simulink model "dynamic_simulation"  (R2020a)
settings: Solver=ode3  StartTime=0.0  StopTime=inf  FixedStep=0.01  RelTol=1e-3
undefined symbols (not defined in the file): name_max_length
libraries: robotlib x23, robotmaniplib x1
settings Model: Creator=ROS_PO  LastModifiedBy=paolo
settings OptimizationCC: EnhancedBackFolding=on  PassReuseOutputArgsAs=Individual arguments  ZeroExternalMemoryAtStartup=off  ZeroInternalMemoryAtStartup=off  MaxStackSize=64  OptimizeBlockOrder=speed  DifferentSizesBufferReuse=on  OptimizationCustomize=off  EfficientTunableParamExpr=on
settings DebuggingCC: ParameterTunabilityLossMsg=error
settings HardwareCC: ProdBitPerPointer=32  ProdBitPerSizeT=32  ProdBitPerPtrDiffT=32  ProdLargestAtomicFloat=None  ProdIntDivRoundTo=Undefined  ProdEndianess=Unspecified  ProdWordSize=32  ProdHWDeviceType=Generic->Unspecified (assume 32-bit Generic)
settings RTWCC: SystemTargetFile=ert.tlc  HardwareBoard=Robot Operating System (ROS)  TemplateMakefile=ert_default_tmf  GenerateReport=on  Toolchain=Catkin  IncludeHyperlinkInReport=on  LaunchReport=on  TargetLang=C++  GenerateTraceInfo=on  GenerateTraceReport=on  GenerateTraceReportSl=on  GenerateTraceReportSf=on  GenerateTraceReportEml=on
settings CodeAppCC: ForceParamTrailComments=on  IgnoreCustomStorageClasses=off  OperatorAnnotations=on  SimulinkDataObjDesc=on  SFDataObjDesc=on  InsertBlockDesc=on
settings ERTTargetCC: SupportContinuousTime=on  SupportVariableSizeSignals=on

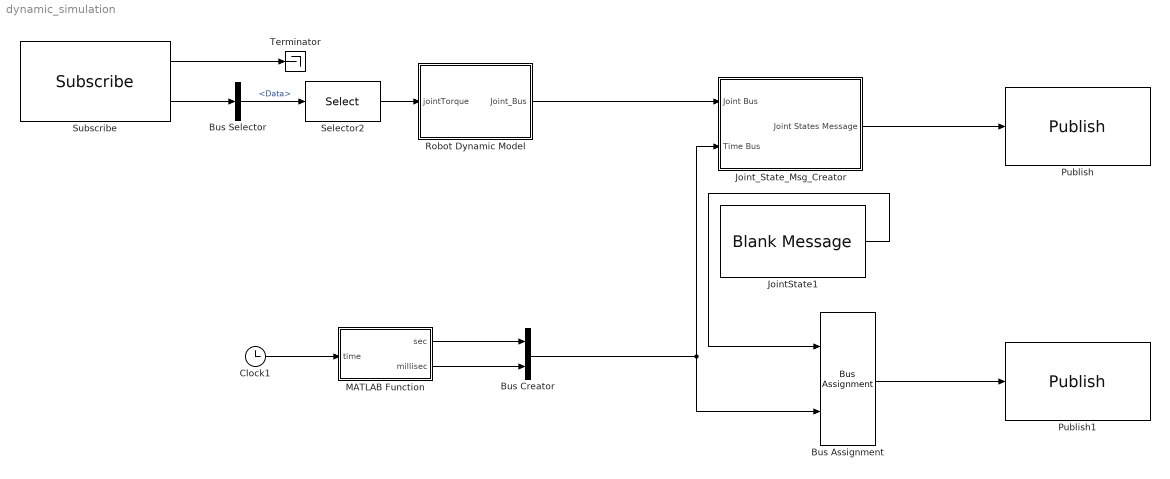
== system dynamic_simulation ==
  Bus Assignment : BusAssignment  AssignedSignals=Clock_
  Bus Creator : BusCreator  Inputs=2
  Bus Selector : BusSelector  OutputSignals=Data
  Clock1 : Clock
  JointState1 : robotlib/Blank Message  messageClass=Message  entityType=rosgraph_msgs/Clock  messageType=rosgraph_msgs/Clock  SampleTime=inf
  Joint_State_Msg_Creator : Subsystem
  MATLAB Function : MATLAB Function  TreatAsAtomicUnit=on
  Publish : robotlib/Publish  topicSource=Specify your own  topic=/joint_states  messageType=sensor_msgs/JointState  messageQueueLength=1
  Publish1 : robotlib/Publish  topicSource=Specify your own  topic=/clock  messageType=rosgraph_msgs/Clock  messageQueueLength=1
  Robot Dynamic Model : Subsystem
  Selector2 : Selector  IndexOptions=Starting index (dialog)  Indices=1  OutputSizes=6
  Subscribe : robotlib/Subscribe  topicSource=Specify your own  topic=/joint_torque  messageType=std_msgs/Float64MultiArray  sampleTime=-1  messageQueueLength=1
  Terminator : Terminator
  wires:
  Subscribe/1 -> Terminator/1
  Subscribe/2 -> Bus Selector/1
  Robot Dynamic Model/1(Joint_Bus) -> Joint_State_Msg_Creator/1(Joint Bus)
  Bus Selector/1 -> Selector2/1  "<Data>"
  MATLAB Function/1(sec) -> Bus Creator/1
  MATLAB Function/2(millisec) -> Bus Creator/2
  Clock1/1 -> MATLAB Function/1(time)
  Bus Creator/1 -> Bus Assignment/2, Joint_State_Msg_Creator/2(Time Bus)
  JointState1/1 -> Bus Assignment/1
  Bus Assignment/1 -> Publish1/1
  Joint_State_Msg_Creator/1(Joint States Message) -> Publish/1
  Selector2/1 -> Robot Dynamic Model/1(jointTorque)

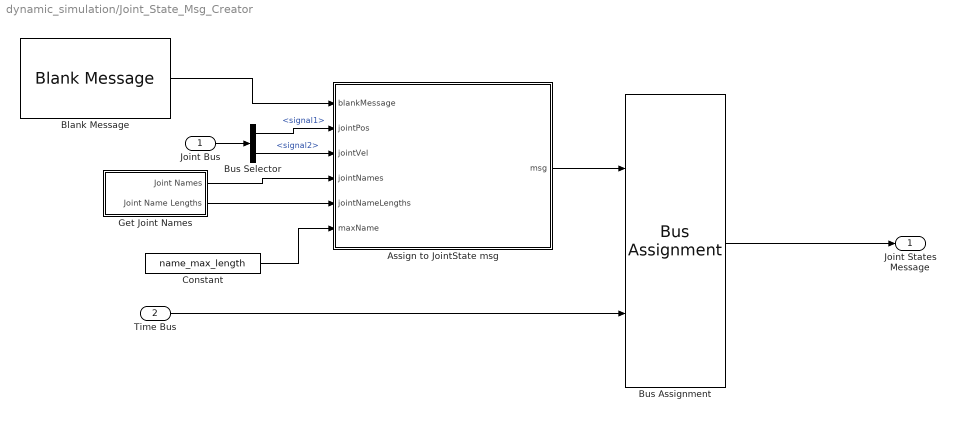
== system dynamic_simulation/Joint_State_Msg_Creator ==
  Joint Bus : Inport
  Time Bus : Inport  Port=2
  Assign to JointState msg : MATLAB Function  TreatAsAtomicUnit=on
  Blank Message : robotlib/Blank Message  messageClass=Message  entityType=sensor_msgs/JointState  messageType=sensor_msgs/JointState  SampleTime=inf
  Bus Assignment : BusAssignment  AssignedSignals=Header.Stamp
  Bus Selector : BusSelector  OutputSignals=signal1,signal2
  Constant : Constant  Value=name_max_length
  Get Joint Names : Subsystem
  Joint States Message : Outport
  wires:
  Joint Bus/1 -> Bus Selector/1
  Bus Selector/1 -> Assign to JointState msg/2(jointPos)  "<signal1>"
  Bus Selector/2 -> Assign to JointState msg/3(jointVel)  "<signal2>"
  Time Bus/1 -> Bus Assignment/2
  Bus Assignment/1 -> Joint States Message/1
  Blank Message/1 -> Assign to JointState msg/1(blankMessage)
  Assign to JointState msg/1(msg) -> Bus Assignment/1
  Get Joint Names/1(Joint Names) -> Assign to JointState msg/4(jointNames)
  Get Joint Names/2(Joint Name Lengths) -> Assign to JointState msg/5(jointNameLengths)
  Constant/1 -> Assign to JointState msg/6(maxName)

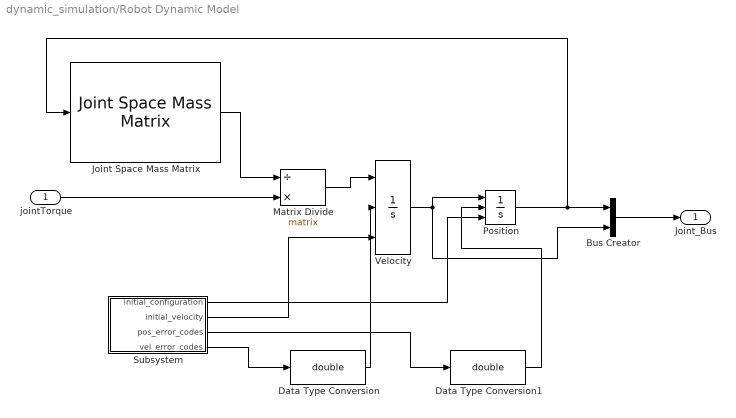
== system dynamic_simulation/Robot Dynamic Model ==
  jointTorque : Inport
  Bus Creator : BusCreator  Inputs=2
  Data Type Conversion : DataTypeConversion  OutDataTypeStr=double
  Data Type Conversion1 : DataTypeConversion  OutDataTypeStr=double
  Joint Space Mass Matrix : robotmaniplib/Joint Space Mass Matrix  RigidBodyTree=robot  SimulateUsing=Interpreted execution
  Matrix Divide : Product  Inputs=/*  Multiplication=Matrix(*)
  Position : Integrator  ExternalReset=falling  InitialConditionSource=external
  Subsystem : Subsystem
  Velocity : Integrator  ExternalReset=falling  InitialConditionSource=external
  Joint_Bus : Outport
  wires:
  Position/1 -> Joint Space Mass Matrix/1, Bus Creator/1
  Velocity/1 -> Position/1, Bus Creator/2
  Bus Creator/1 -> Joint_Bus/1
  Joint Space Mass Matrix/1 -> Matrix Divide/1
  jointTorque/1 -> Matrix Divide/2
  Matrix Divide/1 -> Velocity/1
  Subsystem/4(vel_error_codes) -> Data Type Conversion/1
  Subsystem/3(pos_error_codes) -> Data Type Conversion1/1
  Data Type Conversion/1 -> Velocity/2
  Subsystem/2(initial_velocity) -> Velocity/3
  Data Type Conversion1/1 -> Position/2
  Subsystem/1(initial_configuration) -> Position/3

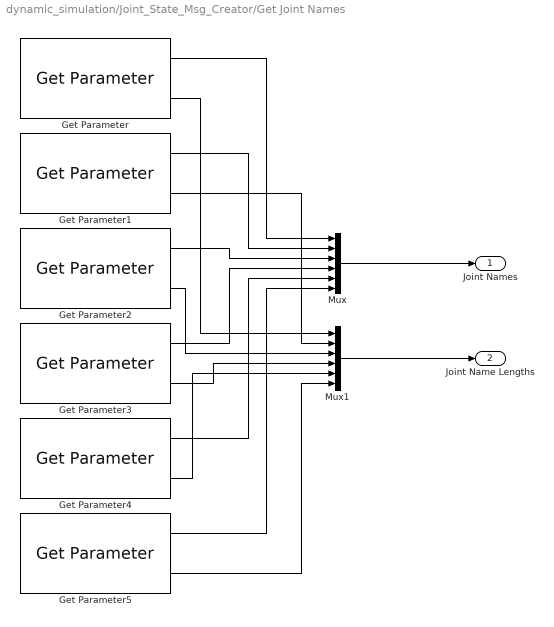
== system dynamic_simulation/Joint_State_Msg_Creator/Get Joint Names ==
  Get Parameter : robotlib/Get Parameter  ParameterSource=Select from ROS network  ParameterName=/controller_joint_name_1  ParameterType=uint8[] (string)  ParameterMaxArrayLength=name_max_length  ParameterInitialValue=default_name_1  SampleTime=-1  ShowErrorCodeOutput=off  ModelName=dynamic_simulation  BlockId=ParamGet_dynamic_simulation_224
      settings: SourceProductBaseCode=RR
  Get Parameter1 : robotlib/Get Parameter  ParameterSource=Specify your own  ParameterName=/controller_joint_name_2  ParameterType=uint8[] (string)  ParameterMaxArrayLength=name_max_length  ParameterInitialValue=default_name_2  SampleTime=-1  ShowErrorCodeOutput=off  ModelName=dynamic_simulation  BlockId=ParamGet_dynamic_simulation_228
      settings: SourceProductBaseCode=RR
  Get Parameter2 : robotlib/Get Parameter  ParameterSource=Specify your own  ParameterName=/controller_joint_name_3  ParameterType=uint8[] (string)  ParameterMaxArrayLength=name_max_length  ParameterInitialValue=default_name_3  SampleTime=-1  ShowErrorCodeOutput=off  ModelName=dynamic_simulation  BlockId=ParamGet_dynamic_simulation_229
      settings: SourceProductBaseCode=RR
  Get Parameter3 : robotlib/Get Parameter  ParameterSource=Specify your own  ParameterName=/controller_joint_name_4  ParameterType=uint8[] (string)  ParameterMaxArrayLength=name_max_length  ParameterInitialValue=default_name_4  SampleTime=-1  ShowErrorCodeOutput=off  ModelName=dynamic_simulation  BlockId=ParamGet_dynamic_simulation_230
      settings: SourceProductBaseCode=RR
  Get Parameter4 : robotlib/Get Parameter  ParameterSource=Specify your own  ParameterName=/controller_joint_name_5  ParameterType=uint8[] (string)  ParameterMaxArrayLength=name_max_length  ParameterInitialValue=default_name_5  SampleTime=-1  ShowErrorCodeOutput=off  ModelName=dynamic_simulation  BlockId=ParamGet_dynamic_simulation_231
      settings: SourceProductBaseCode=RR
  Get Parameter5 : robotlib/Get Parameter  ParameterSource=Specify your own  ParameterName=/controller_joint_name_6  ParameterType=uint8[] (string)  ParameterMaxArrayLength=name_max_length  ParameterInitialValue=default_name_6  SampleTime=-1  ShowErrorCodeOutput=off  ModelName=dynamic_simulation  BlockId=ParamGet_dynamic_simulation_232
      settings: SourceProductBaseCode=RR
  Mux : Mux  Inputs=6
  Mux1 : Mux  Inputs=6
  Joint Names : Outport
  Joint Name Lengths : Outport  Port=2
  wires:
  Get Parameter/1 -> Mux/1
  Get Parameter1/1 -> Mux/2
  Get Parameter2/1 -> Mux/3
  Get Parameter3/1 -> Mux/4
  Get Parameter4/1 -> Mux/5
  Get Parameter5/1 -> Mux/6
  Get Parameter/2 -> Mux1/1
  Get Parameter1/2 -> Mux1/2
  Get Parameter2/2 -> Mux1/3
  Get Parameter3/2 -> Mux1/4
  Get Parameter4/2 -> Mux1/5
  Get Parameter5/2 -> Mux1/6
  Mux/1 -> Joint Names/1
  Mux1/1 -> Joint Name Lengths/1

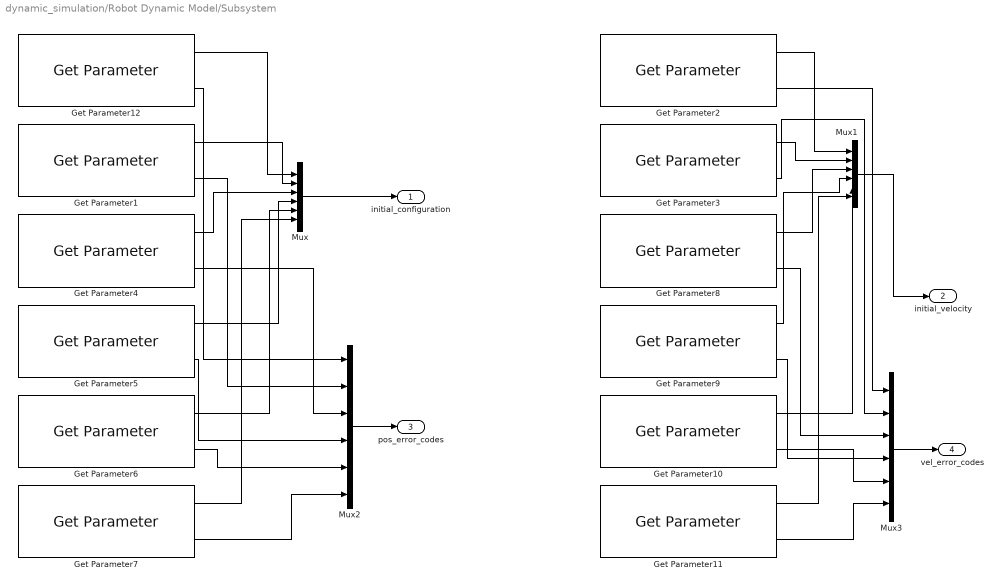
== system dynamic_simulation/Robot Dynamic Model/Subsystem ==
  Get Parameter1 : robotlib/Get Parameter  ParameterSource=Specify your own  ParameterName=/q2_initial  ParameterType=double  ParameterMaxArrayLength=16  ParameterInitialValue=0  SampleTime=-1  ShowErrorCodeOutput=on  ModelName=dynamic_simulation  BlockId=ParamGet_dynamic_simulation_132
      settings: SourceProductBaseCode=RR
  Get Parameter10 : robotlib/Get Parameter  ParameterSource=Specify your own  ParameterName=/qv5_initial  ParameterType=double  ParameterMaxArrayLength=16  ParameterInitialValue=0  SampleTime=-1  ShowErrorCodeOutput=on  ModelName=dynamic_simulation  BlockId=ParamGet_dynamic_simulation_133
      settings: SourceProductBaseCode=RR
  Get Parameter11 : robotlib/Get Parameter  ParameterSource=Specify your own  ParameterName=/qv6_initial  ParameterType=double  ParameterMaxArrayLength=16  ParameterInitialValue=0  SampleTime=-1  ShowErrorCodeOutput=on  ModelName=dynamic_simulation  BlockId=ParamGet_dynamic_simulation_134
      settings: SourceProductBaseCode=RR
  Get Parameter12 : robotlib/Get Parameter  ParameterSource=Specify your own  ParameterName=/q1_initial  ParameterType=double  ParameterMaxArrayLength=16  ParameterInitialValue=0  SampleTime=-1  ShowErrorCodeOutput=on  ModelName=dynamic_simulation  BlockId=ParamGet_dynamic_simulation_194
      settings: SourceProductBaseCode=RR
  Get Parameter2 : robotlib/Get Parameter  ParameterSource=Specify your own  ParameterName=/qv1_initial  ParameterType=double  ParameterMaxArrayLength=16  ParameterInitialValue=0  SampleTime=-1  ShowErrorCodeOutput=on  ModelName=dynamic_simulation  BlockId=ParamGet_dynamic_simulation_135
      settings: SourceProductBaseCode=RR
  Get Parameter3 : robotlib/Get Parameter  ParameterSource=Specify your own  ParameterName=/qv2_initial  ParameterType=double  ParameterMaxArrayLength=16  ParameterInitialValue=0  SampleTime=-1  ShowErrorCodeOutput=on  ModelName=dynamic_simulation  BlockId=ParamGet_dynamic_simulation_136
      settings: SourceProductBaseCode=RR
  Get Parameter4 : robotlib/Get Parameter  ParameterSource=Specify your own  ParameterName=/q3_initial  ParameterType=double  ParameterMaxArrayLength=16  ParameterInitialValue=0  SampleTime=-1  ShowErrorCodeOutput=on  ModelName=dynamic_simulation  BlockId=ParamGet_dynamic_simulation_137
      settings: SourceProductBaseCode=RR
  Get Parameter5 : robotlib/Get Parameter  ParameterSource=Specify your own  ParameterName=/q4_initial  ParameterType=double  ParameterMaxArrayLength=16  ParameterInitialValue=0  SampleTime=-1  ShowErrorCodeOutput=on  ModelName=dynamic_simulation  BlockId=ParamGet_dynamic_simulation_138
      settings: SourceProductBaseCode=RR
  Get Parameter6 : robotlib/Get Parameter  ParameterSource=Specify your own  ParameterName=/q5_initial  ParameterType=double  ParameterMaxArrayLength=16  ParameterInitialValue=0  SampleTime=-1  ShowErrorCodeOutput=on  ModelName=dynamic_simulation  BlockId=ParamGet_dynamic_simulation_139
      settings: SourceProductBaseCode=RR
  Get Parameter7 : robotlib/Get Parameter  ParameterSource=Specify your own  ParameterName=/q6_initial  ParameterType=double  ParameterMaxArrayLength=16  ParameterInitialValue=0  SampleTime=-1  ShowErrorCodeOutput=on  ModelName=dynamic_simulation  BlockId=ParamGet_dynamic_simulation_140
      settings: SourceProductBaseCode=RR
  Get Parameter8 : robotlib/Get Parameter  ParameterSource=Specify your own  ParameterName=/qv3_initial  ParameterType=double  ParameterMaxArrayLength=16  ParameterInitialValue=0  SampleTime=-1  ShowErrorCodeOutput=on  ModelName=dynamic_simulation  BlockId=ParamGet_dynamic_simulation_141
      settings: SourceProductBaseCode=RR
  Get Parameter9 : robotlib/Get Parameter  ParameterSource=Specify your own  ParameterName=/qv4_initial  ParameterType=double  ParameterMaxArrayLength=16  ParameterInitialValue=0  SampleTime=-1  ShowErrorCodeOutput=on  ModelName=dynamic_simulation  BlockId=ParamGet_dynamic_simulation_142
      settings: SourceProductBaseCode=RR
  Mux{,1..3} (4 alike) : Mux  Inputs=6
  initial_configuration : Outport
  initial_velocity : Outport  Port=2
  pos_error_codes : Outport  Port=3
  vel_error_codes : Outport  Port=4
  wires:
  Mux/1 -> initial_configuration/1
  Get Parameter12/1 -> Mux/1
  Get Parameter1/1 -> Mux/2
  Get Parameter3/1 -> Mux1/2
  Get Parameter2/1 -> Mux1/1
  Mux1/1 -> initial_velocity/1
  Get Parameter4/1 -> Mux/3
  Get Parameter5/1 -> Mux/4
  Get Parameter6/1 -> Mux/5
  Get Parameter7/1 -> Mux/6
  Get Parameter8/1 -> Mux1/3
  Get Parameter9/1 -> Mux1/4
  Get Parameter10/1 -> Mux1/5
  Get Parameter12/2 -> Mux2/1
  Get Parameter1/2 -> Mux2/2
  Get Parameter4/2 -> Mux2/3
  Get Parameter5/2 -> Mux2/4
  Get Parameter6/2 -> Mux2/5
  Get Parameter7/2 -> Mux2/6
  Mux2/1 -> pos_error_codes/1
  Get Parameter11/1 -> Mux1/6
  Get Parameter2/2 -> Mux3/1
  Get Parameter3/2 -> Mux3/2
  Get Parameter8/2 -> Mux3/3
  Get Parameter9/2 -> Mux3/4
  Get Parameter10/2 -> Mux3/5
  Get Parameter11/2 -> Mux3/6
  Mux3/1 -> vel_error_codes/1

== matlab function dynamic_simulation/MATLAB Function ==
  data: time input; sec output; millisec output
function [sec, millisec] = fcn(time)

    sec = fix(time);
    millisec = fix((time - fix(time)) * 1e9);

== matlab function dynamic_simulation/Joint_State_Msg_Creator/Assign to JointState msg ==
  data: blankMessage input; msg output Bus: SL_Bus_dynamic_simulation_sensor_msgs_JointState; jointPos input; jointVel input; jointNames input; jointNameLengths input; maxName input
function msg = assign_JointState(blankMessage, jointPos, jointVel, jointNames, jointNameLengths, maxName)
%#codegen

% Assign the output message to be the same with input blank message
msg = blankMessage;

% Initialize time stamp


% Set the number of strings in the string array, and joint positions/velocities in the position/velocity array
numJoints = length(jointPos);
msg.Name_SL_Info.CurrentLength = uint32(numJoints);
msg.Position_SL_Info.CurrentLength = uint32(numJoints);
msg.Velocity_SL_Info.CurrentLength = uint32(numJoints);

% Set the individual components in the message arrays

for idx=1:numJoints
    
    start = uint32((idx - 1) * maxName + 1);
    
    msg.Name(idx).Data(1:jointNameLengths(idx)) = jointNames(start:start+jointNameLengths(idx)-1);
    msg.Name(idx).Data_SL_Info.CurrentLength = jointNameLengths(idx);
    
    msg.Position(idx) = jointPos(idx);
    msg.Velocity(idx) = jointVel(idx);
    
end
